simulink model "pendule_inverse"  (R2015a)
settings: Solver=ode3  StartTime=0.0  StopTime=10.0  FixedStep=0.01  RelTol=1e-3
undefined symbols (not defined in the file): l
libraries: simulink x1
settings Model: Creator=fschalle  LastModifiedBy=root

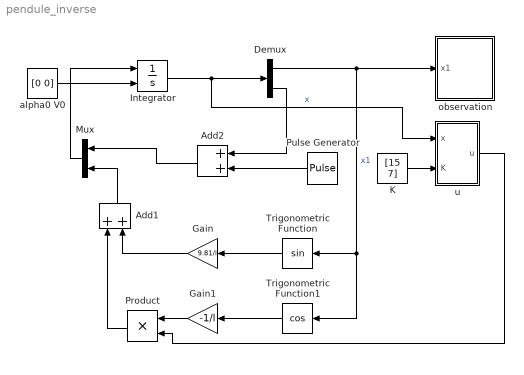
== system pendule_inverse ==
  Add1 : Sum
  Add2 : Sum
  Demux : Demux  Outputs=2
  Gain : Gain  Gain=9.81/l
  Gain1 : Gain  Gain=-1/l
  Integrator : Integrator  InitialConditionSource=external
  "K " : Constant  Value=[15 7]
  Mux : Mux  Inputs=2
  Product : Product
  Pulse Generator : DiscretePulseGenerator  PulseType=Time based  Period=10  PulseWidth=5  PhaseDelay=1
  Trigonometric Function : Trigonometry
  Trigonometric Function1 : Trigonometry  Operator=cos
  alpha0 V0 : Constant  Value=[0 0]
  observation : Subsystem
  u : Subsystem
  wires:
  alpha0 V0/1 -> Integrator/2
  Integrator/1 -> u/1(x), Demux/1  "x"
  Mux/1 -> Integrator/1
  Trigonometric Function/1 -> Gain/1
  Demux/1 -> Trigonometric Function1/1, Trigonometric Function/1, observation/1(x1)  "x1"
  Add1/1 -> Mux/2
  Gain/1 -> Add1/2
  Trigonometric Function1/1 -> Gain1/1
  Gain1/1 -> Product/1
  Product/1 -> Add1/1
  Add2/1 -> Mux/1
  Pulse Generator/1 -> Add2/2
  Demux/2 -> Add2/1
  "K "/1 -> u/2(K)
  u/1(u) -> Product/2

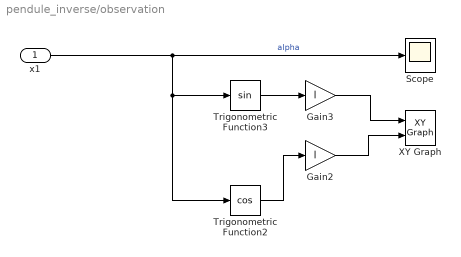
== system pendule_inverse/observation ==
  x1 : Inport
  Gain2 : Gain  Gain=l
  Gain3 : Gain  Gain=l
  Scope : Scope
      settings: YMin=0  YMax=0.425
  Trigonometric Function2 : Trigonometry  Operator=cos
  Trigonometric Function3 : Trigonometry
  XY Graph : simulink/Sinks/XY Graph  xmin=-0.1  xmax=0.1  ymin=-0.1  ymax=0.1  st=-1
  wires:
  Trigonometric Function3/1 -> Gain3/1
  Trigonometric Function2/1 -> Gain2/1
  Gain2/1 -> XY Graph/2
  x1/1 -> Scope/1, Trigonometric Function2/1, Trigonometric Function3/1  "alpha"
  Gain3/1 -> XY Graph/1

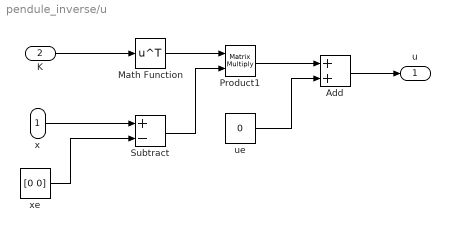
== system pendule_inverse/u ==
  x : Inport
  K : Inport  Port=2
  Add : Sum
  Math Function : Math  Operator=transpose  SaturateOnIntegerOverflow=on
  Product1 : Product  Multiplication=Matrix(*)
  Subtract : Sum  Inputs=+-
  ue : Constant  Value=0
  xe : Constant  Value=[0 0]
  u : Outport
  wires:
  K/1 -> Math Function/1
  xe/1 -> Subtract/2
  Add/1 -> u/1
  Product1/1 -> Add/1
  ue/1 -> Add/2
  Math Function/1 -> Product1/1
  Subtract/1 -> Product1/2
  x/1 -> Subtract/1
